simulink model "Simulink_model"  (R2024b)
settings: Solver=FixedStepAuto  StartTime=0.0  StopTime=10.0  FixedStep=1e-3  RelTol=1e-3
values from neighbouring files (symbols this model uses):
  C = [1 0]    [Script.m]
undefined symbols (not defined in the file or in its folder): G
settings Model: Creator=Enrico  LastModifiedBy=Enrico

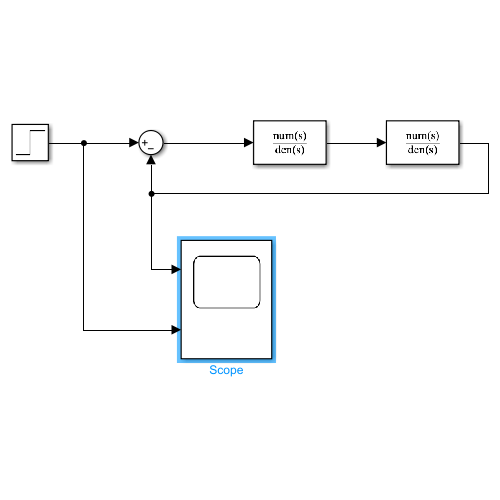
[thumbnail: Simulink's stored preview of the top-level diagram]
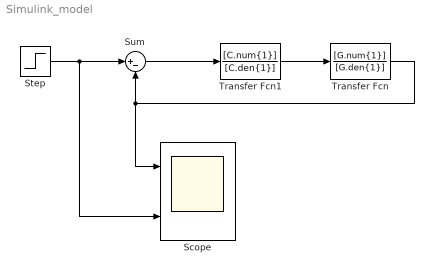
== system Simulink_model ==
  Scope : Scope  NumInputPorts=2
  Step : Step  SampleTime=0
  Sum : Sum  Inputs=|+-
  Transfer Fcn : TransferFcn  Numerator=[G.num{1}]  Denominator=[G.den{1}]
  Transfer Fcn1 : TransferFcn  Numerator=[C.num{1}]  Denominator=[C.den{1}]
  wires:
  Transfer Fcn1/1 -> Transfer Fcn/1
  Sum/1 -> Transfer Fcn1/1
  Transfer Fcn/1 -> Scope/1, Sum/2
  Step/1 -> Scope/2, Sum/1
